simulink model "2025-11-18 - V0.2.6 - FullFMS"  (R2025b)
settings: Solver=VariableStepAuto  StartTime=0.0  StopTime=inf  RelTol=1e-3
libraries: opcualib x8
(part 1 of 3)
settings Model: SimulationMode=accelerator  Creator=guilh  LastModifiedBy=guilh

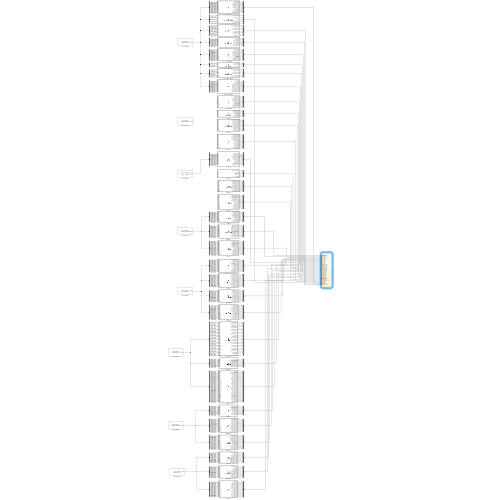
[thumbnail: Simulink's stored preview of the top-level diagram]
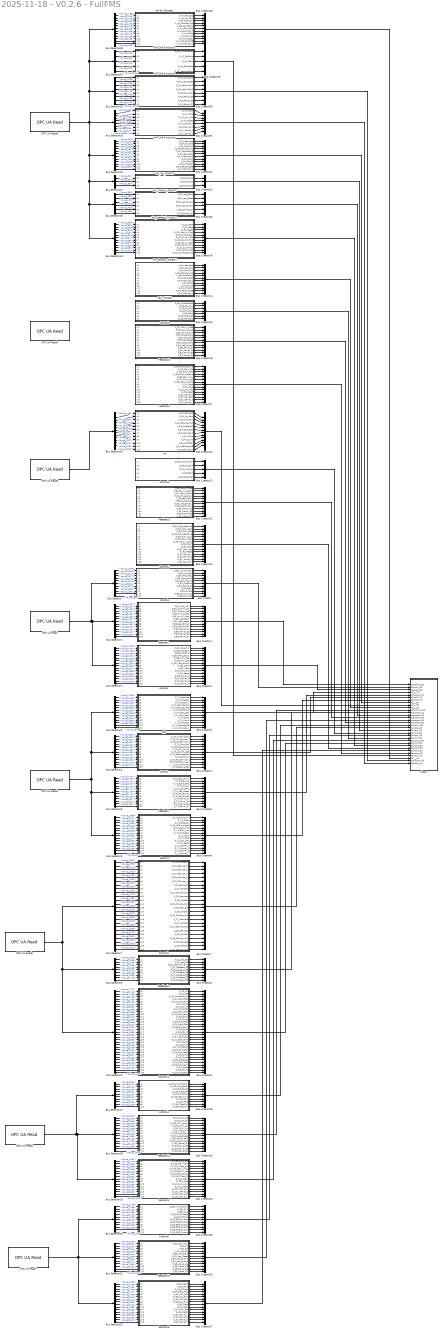
== system 2025-11-18 - V0.2.6 - FullFMS ==
  ASI : MATLAB Function  TreatAsAtomicUnit=on
  Asi : MATLAB Function  TreatAsAtomicUnit=on
  Asi1_HAND2 : MATLAB Function  TreatAsAtomicUnit=on
  Bus Creator : BusCreator  Inputs=11
  Bus Creator1 : BusCreator  Inputs=13
  Bus Creator{5,10,12,14,16,21,24,26,28} (9 alike) : BusCreator  Inputs=12
  Bus Creator11 : BusCreator  Inputs=5
  Bus Creator{2,6,13,17,20} (5 alike) : BusCreator  Inputs=15
  Bus Creator15 : BusCreator  Inputs=7
  Bus Creator18 : BusCreator  Inputs=10
  Bus Creator19 : BusCreator  Inputs=14
  Bus Creator22 : BusCreator  Inputs=3
  Bus Creator23 : BusCreator  Inputs=6
  Bus Creator25 : BusCreator  Inputs=11
  Bus Creator27 : BusCreator  Inputs=16
  Bus Creator29 : BusCreator  Inputs=5
  Bus Creator3 : BusCreator  Inputs=13
  Bus Creator30 : BusCreator  Inputs=8
  Bus Creator31 : BusCreator  Inputs=8
  Bus Creator4 : BusCreator  Inputs=13
  Bus Creator7 : BusCreator  Inputs=24
  Bus Creator8 : BusCreator  Inputs=9
  Bus Creator9 : BusCreator  Inputs=33
  Bus Selector : BusSelector  OutputSignals=Value_1195,Value_1205,Value_1215,Value_1227,Value_1239,Value_1249,Value_1261,Value_1271,Value_1281,Value_1291,Value_1301
  Bus Selector1 : BusSelector  OutputSignals=Value_1317,Value_1327,Value_1337,Value_1347,Value_1357,Value_1367,Value_1377,Value_1387,Value_1397,Value_1407,Value_1417,Value_1427,Value_1437
  Bus Selector10 : BusSelector  OutputSignals=Value_1457,Value_1467,Value_1477,Value_1487,Value_1497,Value_1507,Value_1517,Value_1527,Value_1537,Value_1547,Value_1557,Value_1567
  Bus Selector16 : BusSelector  OutputSignals=Value_215,Value_225,Value_235,Value_245,Value_255,Value_265,Value_275,Value_285,Value_295,Value_305,Value_315,Value_325
  Bus Selector17 : BusSelector  OutputSignals=Value_341,Value_354,Value_367
  Bus Selector18 : BusSelector  OutputSignals=Value_383,Value_393,Value_403,Value_413,Value_423,Value_433
  Bus Selector19 : BusSelector  OutputSignals=Value_569,Value_582,Value_595,Value_608,Value_621,Value_634,Value_647,Value_660,Value_673,Value_686,Value_699,Value_712
  Bus Selector2 : BusSelector  OutputSignals=Value_1458,Value_1471,Value_1486,Value_1499,Value_1512,Value_1525,Value_1538,Value_1551,Value_1564,Value_1577,Value_1590,Value_1603,Value_1616,Value_1629,Value_1642
  Bus Selector20 : BusSelector  OutputSignals=Value_1178,Value_1188,Value_1198,Value_1208,Value_1218,Value_1228,Value_1238,Value_1248,Value_1258,Value_1268,Value_1278
  Bus Selector21 : BusSelector  OutputSignals=Value_1294,Value_1304,Value_1314,Value_1324,Value_1334,Value_1344,Value_1354,Value_1364,Value_1374,Value_1384,Value_1394,Value_1404
  Bus Selector22 : BusSelector  OutputSignals=Value_1423,Value_1436,Value_1451,Value_1464,Value_1477,Value_1490,Value_1503,Value_1516,Value_1529,Value_1542,Value_1555,Value_1568,Value_1581,Value_1594,Value_1607,Value_1620
  Bus Selector23 : BusSelector  OutputSignals=Value_1198,Value_1208,Value_1218,Value_1228,Value_1238,Value_1248,Value_1258,Value_1268,Value_1278,Value_1288,Value_1298,Value_1308
  Bus Selector24 : BusSelector  OutputSignals=Value_1324,Value_1334,Value_1344,Value_1354,Value_1364
  Bus Selector25 : BusSelector  OutputSignals=Value_1380,Value_1390,Value_1400,Value_1410,Value_1420,Value_1430,Value_1440,Value_1450
  Bus Selector26 : BusSelector  OutputSignals=Value_1469,Value_1482,Value_1495,Value_1508,Value_1521,Value_1534,Value_1547,Value_1560
  Bus Selector27 : BusSelector  OutputSignals=Value_1204,Value_1214,Value_1224,Value_1234,Value_1244,Value_1254,Value_1264,Value_1274,Value_1284,Value_1294
  Bus Selector28 : BusSelector  OutputSignals=Value_1310,Value_1320,Value_1330,Value_1340,Value_1350,Value_1360,Value_1370,Value_1380,Value_1390,Value_1400,Value_1410,Value_1420,Value_1430,Value_1440
  Bus Selector29 : BusSelector  OutputSignals=Value_1461,Value_1474,Value_1489,Value_1502,Value_1515,Value_1528,Value_1541,Value_1554,Value_1567,Value_1580,Value_1593,Value_1606,Value_1619,Value_1632,Value_1645
  Bus Selector3 : BusSelector  OutputSignals=Value_1455,Value_1465,Value_1475,Value_1485,Value_1495,Value_1505,Value_1515,Value_1525,Value_1535,Value_1545,Value_1555,Value_1565,Value_1575
  Bus Selector4 : BusSelector  OutputSignals=Value_1591,Value_1601,Value_1611,Value_1621,Value_1631,Value_1641,Value_1651,Value_1661,Value_1671,Value_1681,Value_1691,Value_1701,Value_1711
  Bus Selector5 : BusSelector  OutputSignals=Value_1727,Value_1737,Value_1747,Value_1757,Value_1767,Value_1777,Value_1787,Value_1797,Value_1807,Value_1817,Value_1827,Value_1837
  Bus Selector6 : BusSelector  OutputSignals=Value_1858,Value_1871,Value_1886,Value_1899,Value_1912,Value_1925,Value_1938,Value_1951,Value_1964,Value_1977,Value_1990,Value_2003,Value_2016,Value_2029,Value_2042
  Bus Selector7 : BusSelector  OutputSignals=Value_1382,Value_1392,Value_1402,Value_1412,Value_1422,Value_1432,Value_1442,Value_1452,Value_1462,Value_1472,Value_1482,Value_1492,Value_1502,Value_1512,Value_1522,Value_1532,Value_1542,Value_1552,Value_1562,Value_1572,Value_1582,Value_1592,Value_1602,Value_1612
  Bus Selector8 : BusSelector  OutputSignals=Value_1628,Value_1638,Value_1648,Value_1658,Value_1668,Value_1678,Value_1688,Value_1698,Value_1708
  Bus Selector9 : BusSelector  OutputSignals=Value_1727,Value_1740,Value_1755,Value_1768,Value_1781,Value_1794,Value_1807,Value_1820,Value_1833,Value_1846,Value_1859,Value_1872,Value_1885,Value_1898,Value_1911,Value_1924,Value_1937,Value_1950,Value_1963,Value_1976,Value_1989,Value_2002,Value_2015,Value_2028,Value_2041,Value_2054,Value_2067,Value_2080,Value_2093,Value_2106,Value_2119,Value_2132,Value_2145
  Chart : Stateflow chart  TreatAsAtomicUnit=on
      settings: PortSchema="{\"entries\":[{\"content\":{\"sides\":[{\"content\":{\"connectorIds\":[\"In2\",\"In1\",\"In3\",\"In4\",\"In6\",\"In5\",\"In7\",\"In8\",\"In9\",\"In10\",\"In11\",\"In12\",\"In13\",\"In14\",\"In15\",\"In16\",\"In17\",\"In18\",\"In19\",\"In20\",\"In21\",\"In22\",\"In23\",\"In24\",\"In25\",\"In26\",\"In27\",\"In28\",\"In29\",\"In30\",\"In31\",\"In32\"]},\"type\":\"ConnectorPlacement.EquallySpacedRectSide\",\"uuid\":\"e54bf7d4-7c7d-41d9-a8b8-f479ac319a99\"},{\"content\":{\"side\":\"RIGHT\"},\"type\":\"ConnectorPlacement.EquallySpacedRectSide\",\"uuid\":\"d3c20706-71bd-4e26-b40f-0ee7e71b06ee\"},{\"content\":{\"side\":\"TOP\"},\"type\":\"ConnectorPlacement.EquallySpacedRectSide\",\"uuid\":\"ecfb6920-e95b-4ed8-99f9-df5ce878328e\"}]},\"type\":\"ConnectorPlacement.EquallySpacedConnector\",\"uuid\":\"2e714192-4eea-4e1a-8945-7c827feed48f\"}],\"packageUris\":[\"http://schema.mathworks.com/mf0/Connector/R2020b\"],\"version\":\"1.0\"}"
  Control : MATLAB Function  TreatAsAtomicUnit=on
  Control1 : MATLAB Function  TreatAsAtomicUnit=on
  Control2 : MATLAB Function  TreatAsAtomicUnit=on
  Control3 : MATLAB Function  TreatAsAtomicUnit=on
  Control4 : MATLAB Function  TreatAsAtomicUnit=on
  Control5 : MATLAB Function  TreatAsAtomicUnit=on
  Feedback : MATLAB Function  TreatAsAtomicUnit=on
  Feedback1 : MATLAB Function  TreatAsAtomicUnit=on
  Feedback2 : MATLAB Function  TreatAsAtomicUnit=on
  Feedback3 : MATLAB Function  TreatAsAtomicUnit=on
  Feedback4 : MATLAB Function  TreatAsAtomicUnit=on
  Feedback5 : MATLAB Function  TreatAsAtomicUnit=on
  MATLAB Function1 : MATLAB Function  TreatAsAtomicUnit=on
  MATLAB Function2 : MATLAB Function  TreatAsAtomicUnit=on
  MATLAB Function3 : MATLAB Function  TreatAsAtomicUnit=on
  OPC UA Read : opcualib/OPC UA Read  SelectedServer=AAS OPC Distribution  ServerList=AAS OPC Distribution  NodeList={ '1', 'Value', '6', '1195', '1'; '2', 'Value', '6', '1205', '1'; '3', 'Value', '6', '1215', '1'; '4', 'Value', '6', '1227', '1'; '5', 'Value', '6', '1239', '1'; '6', 'Value', '6', '1249', '1'; '7', 'Value', '6', '1261', '1'; '8', 'Value', '6', '1271', '1'; '9', 'Value', '6', '1281', '1'; '10', 'Value', '6', '1291', '1'; '11', 'Value', '6', '1301', '1'; '12', 'Value', '6', '1317', '1'; '13', 'Value', '6', '1327', '1'; '14', 'Value', '6', '1337', '1'; '15', 'Value', '6', '1347', '1'; '16', 'Value', '6', '1357', '1'; '17', 'Value', '6', '1367', '1'; '18', 'Value', '6', '1377', '1'; '19', 'Value', '6', '1387', '1'; '20', 'Value', '6', '1397', '1'; '21', 'Value', '6', '1407', '1'; '22', 'Value', '6', '1417', '1'; '23', 'Value', '6', '1427', '1'; '24', 'Value', '6', '1437', '1'; '25', 'Value', '6', '1458', '1'; '26', 'Value', '6', '1471', '1'; '27', 'Value', '6', '1486', '1'; '28', 'Value', '6', '1499', '1'; '29', 'Value', '6', '1512', '1'; '30', 'Value', '6', '1525', '1'; '31', 'Value', '6', '1538', '1'; '32', 'Value', '6', '1551', '1'; '33', 'Value', '6', '1564', '1'; '34', 'Value', '6', '1577', '1'; '35', 'Value', '6', '1590', '1'; '36', 'Value', '6', '1603', '1'; '37', 'Value', '6', '1616', '1'; '38', 'Value', '6', '1629', '1'; '39', 'Value', '6', '1642', '1' }  ShowQualityPort=off  ShowTimestampPort=off  ShowTimestampPortAs=Seconds since start  SampleTime=-1
  OPC UA Read1 : opcualib/OPC UA Read  SelectedServer=AAS OPC Testing  ServerList=AAS OPC Testing  NodeList={ '1', 'Value', '6', '1455', '1'; '2', 'Value', '6', '1465', '1'; '3', 'Value', '6', '1475', '1'; '4', 'Value', '6', '1485', '1'; '5', 'Value', '6', '1495', '1'; '6', 'Value', '6', '1505', '1'; '7', 'Value', '6', '1515', '1'; '8', 'Value', '6', '1525', '1'; '9', 'Value', '6', '1535', '1'; '10', 'Value', '6', '1545', '1'; '11', 'Value', '6', '1555', '1'; '12', 'Value', '6', '1565', '1'; '13', 'Value', '6', '1575', '1'; '14', 'Value', '6', '1591', '1'; '15', 'Value', '6', '1601', '1'; '16', 'Value', '6', '1611', '1'; '17', 'Value', '6', '1621', '1'; '18', 'Value', '6', '1631', '1'; '19', 'Value', '6', '1641', '1'; '20', 'Value', '6', '1651', '1'; '21', 'Value', '6', '1661', '1'; '22', 'Value', '6', '1671', '1'; '23', 'Value', '6', '1681', '1'; '24', 'Value', '6', '1691', '1'; '25', 'Value', '6', '1701', '1'; '26', 'Value', '6', '1711', '1'; '27', 'Value', '6', '1727', '1'; '28', 'Value', '6', '1737', '1'; '29', 'Value', '6', '1747', '1'; '30', 'Value', '6', '1757', '1'; '31', 'Value', '6', '1767', '1'; '32', 'Value', '6', '1777', '1'; '33', 'Value', '6', '1787', '1'; '34', 'Value', '6', '1797', '1'; '35', 'Value', '6', '1807', '1'; '36', 'Value', '6', '1817', '1'; '37', 'Value', '6', '1827', '1'; '38', 'Value', '6', '1837', '1'; '39', 'Value', '6', '1858', '1'; '40', 'Value', '6', '1871', '1'; '41', 'Value', '6', '1886', '1'; '42', 'Value', '6', '1899', '1'; '43', 'Value', '6', '1912', '1'; '44', 'Value', '6', '1925', '1'; '45', 'Value', '6', '1938', '1'; '46', 'Value', '6', '1951', '1'; '47', 'Value', '6', '1964', '1'; '48', 'Value', '6', '1977', '1'; '49', 'Value', '6', '1990', '1'; '50', 'Value', '6', '2003', '1'; '51', 'Value', '6', '2016', '1'; '52', 'Value', '6', '2029', '1'; '53', 'Value', '6', '2042', '1' }  ShowQualityPort=off  ShowTimestampPort=off  ShowTimestampPortAs=Seconds since start  SampleTime=-1
  OPC UA Read2 : opcualib/OPC UA Read  SelectedServer=AAS OPC Master  ServerList=AAS OPC Master  NodeList={ '1', 'Value', '6', '1382', '1'; '2', 'Value', '6', '1392', '1'; '3', 'Value', '6', '1402', '1'; '4', 'Value', '6', '1412', '1'; '5', 'Value', '6', '1422', '1'; '6', 'Value', '6', '1432', '1'; '7', 'Value', '6', '1442', '1'; '8', 'Value', '6', '1452', '1'; '9', 'Value', '6', '1462', '1'; '10', 'Value', '6', '1472', '1'; '11', 'Value', '6', '1482', '1'; '12', 'Value', '6', '1492', '1'; '13', 'Value', '6', '1502', '1'; '14', 'Value', '6', '1512', '1'; '15', 'Value', '6', '1522', '1'; '16', 'Value', '6', '1532', '1'; '17', 'Value', '6', '1542', '1'; '18', 'Value', '6', '1552', '1'; '19', 'Value', '6', '1562', '1'; '20', 'Value', '6', '1572', '1'; '21', 'Value', '6', '1582', '1'; '22', 'Value', '6', '1592', '1'; '23', 'Value', '6', '1602', '1'; '24', 'Value', '6', '1612', '1'; '25', 'Value', '6', '1628', '1'; '26', 'Value', '6', '1638', '1'; '27', 'Value', '6', '1648', '1'; '28', 'Value', '6', '1658', '1'; '29', 'Value', '6', '1668', '1'; '30', 'Value', '6', '1678', '1'; '31', 'Value', '6', '1688', '1'; '32', 'Value', '6', '1698', '1'; '33', 'Value', '6', '1708', '1'; '34', 'Value', '6', '1727', '1'; '35', 'Value', '6', '1740', '1'; '36', 'Value', '6', '1755', '1'; '37', 'Value', '6', '1768', '1'; '38', 'Value', '6', '1781', '1'; '39', 'Value', '6', '1794', '1'; '40', 'Value', '6', '1807', '1'; '41', 'Value', '6', '1820', '1'; '42', 'Value', '6', '1833', '1'; '43', 'Value', '6', '1846', '1'; '44', 'Value', '6', '1859', '1'; '45', 'Value', '6', '1872', '1'; '46', 'Value', '6', '1885', '1'; '47', 'Value', '6', '1898', '1'; '48', 'Value', '6', '1911', '1'; '49', 'Value', '6', '1924', '1'; '50', 'Value', '6', '1937', '1'; '51', 'Value', '6', '1950', '1'; '52', 'Value', '6', '1963', '1'; '53', 'Value', '6', '1976', '1'; '54', 'Value', '6', '1989', '1'; '55', 'Value', '6', '2002', '1'; '56', 'Value', '6', '2015', '1'; '57', 'Value', '6', '2028', '1'; '58', 'Value', '6', '2041', '1'; '59', 'Value', '6', '2054', '1'; '60', 'Value', '6', '2067', '1'; '61', 'Value', '6', '2080', '1'; '62', 'Value', '6', '2093', '1'; '63', 'Value', '6', '2106', '1'; '64', 'Value', '6', '2119', '1'; '65', 'Value', '6', '2132', '1'; '66', 'Value', '6', '2145', '1' }  ShowQualityPort=off  ShowTimestampPort=off  ShowTimestampPortAs=Seconds since start  SampleTime=-1
  OPC UA Read3 : opcualib/OPC UA Read  SelectedServer=AAS OPC Handling1  ServerList=AAS OPC Handling1  NodeList={ '1', 'Value', '6', '1457', '1'; '2', 'Value', '6', '1467', '1'; '3', 'Value', '6', '1477', '1'; '4', 'Value', '6', '1487', '1'; '5', 'Value', '6', '1497', '1'; '6', 'Value', '6', '1507', '1'; '7', 'Value', '6', '1517', '1'; '8', 'Value', '6', '1527', '1'; '9', 'Value', '6', '1537', '1'; '10', 'Value', '6', '1547', '1'; '11', 'Value', '6', '1557', '1'; '12', 'Value', '6', '1567', '1' }  ShowQualityPort=off  ShowTimestampPort=off  ShowTimestampPortAs=Seconds since start  SampleTime=-1
  OPC UA Read4 : opcualib/OPC UA Read  SelectedServer=AAS OPC Handling2  ServerList=AAS OPC Handling2  NodeList={ '1', 'Value', '6', '572', '1'; '2', 'Value', '6', '582', '1'; '3', 'Value', '6', '592', '1'; '4', 'Value', '6', '602', '1'; '5', 'Value', '6', '612', '1'; '6', 'Value', '6', '622', '1'; '7', 'Value', '6', '632', '1'; '8', 'Value', '6', '642', '1'; '9', 'Value', '6', '652', '1'; '10', 'Value', '6', '662', '1'; '11', 'Value', '6', '672', '1'; '12', 'Value', '6', '682', '1'; '13', 'Value', '6', '698', '1'; '14', 'Value', '6', '708', '1'; '15', 'Value', '6', '718', '1'; '16', 'Value', '6', '728', '1'; '17', 'Value', '6', '738', '1'; '18', 'Value', '6', '748', '1'; '19', 'Value', '6', '758', '1'; '20', 'Value', '6', '774', '1'; '21', 'Value', '6', '784', '1'; '22', 'Value', '6', '794', '1'; '23', 'Value', '6', '804', '1'; '24', 'Value', '6', '814', '1'; '25', 'Value', '6', '824', '1'; '26', 'Value', '6', '834', '1'; '27', 'Value', '6', '844', '1'; '28', 'Value', '6', '854', '1'; '29', 'Value', '6', '864', '1'; '30', 'Value', '6', '874', '1'; '31', 'Value', '6', '884', '1'; '32', 'Value', '6', '905', '1'; '33', 'Value', '6', '918', '1'; '34', 'Value', '6', '933', '1'; '35', 'Value', '6', '946', '1'; '36', 'Value', '6', '959', '1'; '37', 'Value', '6', '972', '1'; '38', 'Value', '6', '985', '1'; '39', 'Value', '6', '998', '1'; '40', 'Value', '6', '1011', '1'; '41', 'Value', '6', '1024', '1'; '42', 'Value', '6', '1037', '1'; '43', 'Value', '6', '1050', '1'; '44', 'Value', '6', '1063', '1'; '45', 'Value', '6', '1076', '1'; '46', 'Value', '6', '1089', '1' }  ShowQualityPort=off  ShowTimestampPort=off  ShowTimestampPortAs=Seconds since start  SampleTime=-1
  OPC UA Read5 : opcualib/OPC UA Read  SelectedServer=AAS OPC Processing  ServerList=AAS OPC Processing  NodeList={ '1', 'Value', '6', '1204', '1'; '2', 'Value', '6', '1214', '1'; '3', 'Value', '6', '1224', '1'; '4', 'Value', '6', '1234', '1'; '5', 'Value', '6', '1244', '1'; '6', 'Value', '6', '1254', '1'; '7', 'Value', '6', '1264', '1'; '8', 'Value', '6', '1274', '1'; '9', 'Value', '6', '1284', '1'; '10', 'Value', '6', '1294', '1'; '11', 'Value', '6', '1310', '1'; '12', 'Value', '6', '1320', '1'; '13', 'Value', '6', '1330', '1'; '14', 'Value', '6', '1340', '1'; '15', 'Value', '6', '1350', '1'; '16', 'Value', '6', '1360', '1'; '17', 'Value', '6', '1370', '1'; '18', 'Value', '6', '1380', '1'; '19', 'Value', '6', '1390', '1'; '20', 'Value', '6', '1400', '1'; '21', 'Value', '6', '1410', '1'; '22', 'Value', '6', '1420', '1'; '23', 'Value', '6', '1430', '1'; '24', 'Value', '6', '1440', '1'; '25', 'Value', '6', '1461', '1'; '26', 'Value', '6', '1474', '1'; '27', 'Value', '6', '1489', '1'; '28', 'Value', '6', '1502', '1'; '29', 'Value', '6', '1515', '1'; '30', 'Value', '6', '1528', '1'; '31', 'Value', '6', '1541', '1'; '32', 'Value', '6', '1554', '1'; '33', 'Value', '6', '1567', '1'; '34', 'Value', '6', '1580', '1'; '35', 'Value', '6', '1593', '1'; '36', 'Value', '6', '1606', '1'; '37', 'Value', '6', '1619', '1'; '38', 'Value', '6', '1632', '1'; '39', 'Value', '6', '1645', '1' }  ShowQualityPort=off  ShowTimestampPort=off  ShowTimestampPortAs=Seconds since start  SampleTime=-1
  OPC UA Read6 : opcualib/OPC UA Read  SelectedServer=Node-RED OPCUA  ServerList=Node-RED OPCUA  NodeList={ '1', 'Value', '6', '215', '1'; '2', 'Value', '6', '225', '1'; '3', 'Value', '6', '235', '1'; '4', 'Value', '6', '245', '1'; '5', 'Value', '6', '255', '1'; '6', 'Value', '6', '265', '1'; '7', 'Value', '6', '275', '1'; '8', 'Value', '6', '285', '1'; '9', 'Value', '6', '295', '1'; '10', 'Value', '6', '305', '1'; '11', 'Value', '6', '315', '1'; '12', 'Value', '6', '325', '1'; '13', 'Value', '6', '341', '1'; '14', 'Value', '6', '354', '1'; '15', 'Value', '6', '367', '1'; '16', 'Value', '6', '383', '1'; '17', 'Value', '6', '393', '1'; '18', 'Value', '6', '403', '1'; '19', 'Value', '6', '413', '1'; '20', 'Value', '6', '423', '1'; '21', 'Value', '6', '433', '1'; '22', 'Value', '6', '569', '1'; '23', 'Value', '6', '582', '1'; '24', 'Value', '6', '595', '1'; '25', 'Value', '6', '608', '1'; '26', 'Value', '6', '621', '1'; '27', 'Value', '6', '634', '1'; '28', 'Value', '6', '647', '1'; '29', 'Value', '6', '660', '1'; '30', 'Value', '6', '673', '1'; '31', 'Value', '6', '686', '1'; '32', 'Value', '6', '699', '1'; '33', 'Value', '6', '712', '1'; '34', 'Value', '6', '1198', '1'; '35', 'Value', '6', '1208', '1'; '36', 'Value', '6', '1218', '1'; '37', 'Value', '6', '1228', '1'; '38', 'Value', '6', '1238', '1'; '39', 'Value', '6', '1248', '1'; '40', 'Value', '6', '1258', '1'; '41', 'Value', '6', '1268', '1'; '42', 'Value', '6', '1278', '1'; '43', 'Value', '6', '1288', '1'; '44', 'Value', '6', '1298', '1'; '45', 'Value', '6', '1308', '1'; '46', 'Value', '6', '1324', '1'; '47', 'Value', '6', '1334', '1'; '48', 'Value', '6', '1344', '1'; '49', 'Value', '6', '1354', '1'; '50', 'Value', '6', '1364', '1'; '51', 'Value', '6', '1380', '1'; '52', 'Value', '6', '1390', '1'; '53', 'Value', '6', '1400', '1'; '54', 'Value', '6', '1410', '1'; '55', 'Value', '6', '1420', '1'; '56', 'Value', '6', '1430', '1'; '57', 'Value', '6', '1440', '1'; '58', 'Value', '6', '1450', '1'; '59', 'Value', '6', '1469', '1'; '60', 'Value', '6', '1482', '1'; '61', 'Value', '6', '1495', '1'; '62', 'Value', '6', '1508', '1'; '63', 'Value', '6', '1521', '1'; '64', 'Value', '6', '1534', '1'; '65', 'Value', '6', '1547', '1'; '66', 'Value', '6', '1560', '1' }  ShowQualityPort=off  ShowTimestampPort=off  ShowTimestampPortAs=Seconds since start  SampleTime=-1
  OPC UA Read7 : opcualib/OPC UA Read  SelectedServer=AAS OPC Sorting  ServerList=AAS OPC Sorting  NodeList={ '1', 'Value', '6', '1178', '1'; '2', 'Value', '6', '1188', '1'; '3', 'Value', '6', '1198', '1'; '4', 'Value', '6', '1208', '1'; '5', 'Value', '6', '1218', '1'; '6', 'Value', '6', '1228', '1'; '7', 'Value', '6', '1238', '1'; '8', 'Value', '6', '1248', '1'; '9', 'Value', '6', '1258', '1'; '10', 'Value', '6', '1268', '1'; '11', 'Value', '6', '1278', '1'; '12', 'Value', '6', '1294', '1'; '13', 'Value', '6', '1304', '1'; '14', 'Value', '6', '1314', '1'; '15', 'Value', '6', '1324', '1'; '16', 'Value', '6', '1334', '1'; '17', 'Value', '6', '1344', '1'; '18', 'Value', '6', '1354', '1'; '19', 'Value', '6', '1364', '1'; '20', 'Value', '6', '1374', '1'; '21', 'Value', '6', '1384', '1'; '22', 'Value', '6', '1394', '1'; '23', 'Value', '6', '1404', '1'; '24', 'Value', '6', '1423', '1'; '25', 'Value', '6', '1436', '1'; '26', 'Value', '6', '1451', '1'; '27', 'Value', '6', '1464', '1'; '28', 'Value', '6', '1477', '1'; '29', 'Value', '6', '1490', '1'; '30', 'Value', '6', '1503', '1'; '31', 'Value', '6', '1516', '1'; '32', 'Value', '6', '1529', '1'; '33', 'Value', '6', '1542', '1'; '34', 'Value', '6', '1555', '1'; '35', 'Value', '6', '1568', '1'; '36', 'Value', '6', '1581', '1'; '37', 'Value', '6', '1594', '1'; '38', 'Value', '6', '1607', '1'; '39', 'Value', '6', '1620', '1' }  ShowQualityPort=off  ShowTimestampPort=off  ShowTimestampPortAs=Seconds since start  SampleTime=-1
  Sensors : MATLAB Function  TreatAsAtomicUnit=on
  Sensors1 : MATLAB Function  TreatAsAtomicUnit=on
  Sensors2 : MATLAB Function  TreatAsAtomicUnit=on
  Sensors3 : MATLAB Function  TreatAsAtomicUnit=on
  Sensors4 : MATLAB Function  TreatAsAtomicUnit=on
  Sensors5 : MATLAB Function  TreatAsAtomicUnit=on
  controls : MATLAB Function  TreatAsAtomicUnit=on
  fcn Asi Storage : MATLAB Function  TreatAsAtomicUnit=on
  fcn_Asi_ROBOT : MATLAB Function  TreatAsAtomicUnit=on
  fcn_Control_ROBOT : MATLAB Function  TreatAsAtomicUnit=on
  fcn_Feedback_ROBOT : MATLAB Function  TreatAsAtomicUnit=on
  fcn_Sensors_ROBOT : MATLAB Function  TreatAsAtomicUnit=on
  feedback : MATLAB Function  TreatAsAtomicUnit=on
  sensors : MATLAB Function  TreatAsAtomicUnit=on
  wires:
  feedback/1(F_82_Pist_Adv) -> Bus Creator1/1
  feedback/2(F_82_Suction_On) -> Bus Creator1/2
  feedback/3(F_82_Suction_Off) -> Bus Creator1/3
  feedback/4(F_82_Arm_2_Del) -> Bus Creator1/4
  feedback/5(F_82_Arm_2_Mag) -> Bus Creator1/5
  feedback/6(F_83_Led_Start) -> Bus Creator1/6
  feedback/7(F_83_Led_Reset) -> Bus Creator1/7
  feedback/8(F_83_Led_Extra1) -> Bus Creator1/8
  feedback/9(F_83_Led_Extra2) -> Bus Creator1/9
  feedback/10(F_83_Panel_O4) -> Bus Creator1/10
  feedback/11(F_83_Panel_O5) -> Bus Creator1/11
  feedback/12(F_83_Panel_O6) -> Bus Creator1/12
  feedback/13(F_83_Panel_O7) -> Bus Creator1/13
  sensors/1(O_80_Mag_Full) -> Bus Creator2/1
  sensors/2(O_80_Pist_Back) -> Bus Creator2/2
  sensors/3(O_80_Pist_Fwd) -> Bus Creator2/3
  sensors/4(O_80_Part_Stuck) -> Bus Creator2/4
  sensors/5(O_80_Arm_Mag) -> Bus Creator2/5
  sensors/6(O_80_Arm_Del) -> Bus Creator2/6
  sensors/7(O_80_Mag_Empty) -> Bus Creator2/7
  sensors/8(O_81_Start) -> Bus Creator2/8
  sensors/9(O_81_Stop) -> Bus Creator2/9
  sensors/10(O_81_Key_Pos) -> Bus Creator2/10
  sensors/11(O_81_Reset) -> Bus Creator2/11
  sensors/12(O_81_Panel_I4) -> Bus Creator2/12
  sensors/13(O_81_Panel_I5) -> Bus Creator2/13
  sensors/14(O_81_Panel_I6) -> Bus Creator2/14
  sensors/15(O_81_Panel_I7) -> Bus Creator2/15
  ASI/1(A_74_Request) -> Bus Creator3/1
  ASI/2(A_74_No_Cart) -> Bus Creator3/2
  ASI/3(A_74_Cart_Full) -> Bus Creator3/3
  ASI/4(A_74_CRoute_Out) -> Bus Creator3/4
  ASI/5(A_74_CRoute_In80) -> Bus Creator3/5
  ASI/6(A_73_TestCartID) -> Bus Creator3/6
  ASI/7(A_74_Cart_Stat) -> Bus Creator3/7
  ASI/8(A_74_Cart_Next) -> Bus Creator3/8
  ASI/9(A_74_Optic) -> Bus Creator3/9
  ASI/10(A_74_Count) -> Bus Creator3/10
  ASI/11(A_74_Pist_Bck) -> Bus Creator3/11
  ASI/12(A_74_Release_FB) -> Bus Creator3/12
  ASI/13(A_74_CRoute_In) -> Bus Creator3/13
  Control/1(C_75_Initialization) -> Bus Creator4/1
  Control/2(C_75_ID_Delivery1) -> Bus Creator4/2
  Control/3(C_75_ID_Delivery2) -> Bus Creator4/3
  Control/4(C_75_Part_Del) -> Bus Creator4/4
  Control/5(C_75_RQ_Part_Del) -> Bus Creator4/5
  Control/6(C_75_RQ_Wrong) -> Bus Creator4/6
  Control/7(C_75_Identified80) -> Bus Creator4/7
  Control/8(C_75_Requested80) -> Bus Creator4/8
  Control/9(C_72_Profibus) -> Bus Creator4/9
  Control/10(C_75_RQ_Delivery1) -> Bus Creator4/10
  Control/11(C_75_RQ_Delivery2) -> Bus Creator4/11
  Control/12(C_75_Identified) -> Bus Creator4/12
  Control/13(C_75_Requested) -> Bus Creator4/13
  Feedback/1(F_72_Elev_Down) -> Bus Creator5/1
  Feedback/2(F_72_Elev_Up) -> Bus Creator5/2
  Feedback/3(F_72_Eject_Part) -> Bus Creator5/3
  Feedback/4(F_72_Air_On) -> Bus Creator5/4
  Feedback/5(F_73_Led_Start) -> Bus Creator5/5
  Feedback/6(F_73_Led_Reset) -> Bus Creator5/6
  Feedback/7(F_73_Led_Extra1) -> Bus Creator5/7
  Feedback/8(F_73_Led_Extra2) -> Bus Creator5/8
  Feedback/9(F_73_Panel_O4) -> Bus Creator5/9
  Feedback/10(F_73_Panel_O5) -> Bus Creator5/10
  Feedback/11(F_73_Panel_O6) -> Bus Creator5/11
  Feedback/12(F_73_Panel_O7) -> Bus Creator5/12
  Sensors/1(O_70_SInductive) -> Bus Creator6/1
  Sensors/2(O_70_SPart) -> Bus Creator6/2
  Sensors/3(O_70_SStation) -> Bus Creator6/3
  Sensors/4(O_70_SPart_Height) -> Bus Creator6/4
  Sensors/5(O_70_Elev_High) -> Bus Creator6/5
  Sensors/6(O_70_Elev_Low) -> Bus Creator6/6
  Sensors/7(O_70_Pist_Back) -> Bus Creator6/7
  Sensors/8(O_71_Start) -> Bus Creator6/8
  Sensors/9(O_71_Stop) -> Bus Creator6/9
  Sensors/10(O_71_Key_Pos) -> Bus Creator6/10
  Sensors/11(O_71_Reset) -> Bus Creator6/11
  Sensors/12(O_71_Panel_I4) -> Bus Creator6/12
  Sensors/13(O_71_Panel_I5) -> Bus Creator6/13
  Sensors/14(O_71_Panel_I6) -> Bus Creator6/14
  Sensors/15(O_71_Panel_I7) -> Bus Creator6/15
  Bus Creator/1 -> Chart/1(Control_80)
  Bus Creator1/1 -> Chart/2(Actuators_80)
  Bus Creator2/1 -> Chart/3(Sensors_80)
  Bus Creator6/1 -> Chart/7(Sensors_70)
  Bus Creator5/1 -> Chart/6(Actuators_70)
  Bus Creator4/1 -> Chart/5(Control_70)
  Bus Creator3/1 -> Chart/4(AS_i_70)
  Control1/1(C_24_CRoute_In) -> Bus Creator7/1
  Control1/2(C_25_CRoute_In) -> Bus Creator7/2
  Control1/3(C_26_CRoute_In) -> Bus Creator7/3
  Control1/4(C_27_CRoute_In) -> Bus Creator7/4
  Control1/5(C_28_CRoute_In) -> Bus Creator7/5
  Control1/6(C_29_CRoute_In) -> Bus Creator7/6
  Control1/7(C_24_Request) -> Bus Creator7/7
  Control1/8(C_24_CartDel) -> Bus Creator7/8
  Control1/9(C_24_CRoute_Out) -> Bus Creator7/9
  Control1/10(C_25_Request) -> Bus Creator7/10
  Control1/11(C_25_CartDel) -> Bus Creator7/11
  Control1/12(C_25_CRoute_Out) -> Bus Creator7/12
  Control1/13(C_26_Request) -> Bus Creator7/13
  Control1/14(C_26_CartDel) -> Bus Creator7/14
  Control1/15(C_26_CRoute_Out) -> Bus Creator7/15
  Control1/16(C_27_Request) -> Bus Creator7/16
  Control1/17(C_27_CartDel) -> Bus Creator7/17
  Control1/18(C_27_CRoute_Out) -> Bus Creator7/18
  Control1/19(C_28_Request) -> Bus Creator7/19
  Control1/20(C_28_CartDel) -> Bus Creator7/20
  Control1/21(C_28_CRoute_Out) -> Bus Creator7/21
  Control1/22(C_29_Request) -> Bus Creator7/22
  Control1/23(C_29_CartDel) -> Bus Creator7/23
  Control1/24(C_29_CRoute_Out) -> Bus Creator7/24
  Feedback1/1(F_22_Led_On) -> Bus Creator8/1
  Feedback1/2(F_22_Led_Off) -> Bus Creator8/2
  Feedback1/3(F_22_Led_Conveyor) -> Bus Creator8/3
  Feedback1/4(F_24_Release_FB) -> Bus Creator8/4
  Feedback1/5(F_25_Release_FB) -> Bus Creator8/5
  Feedback1/6(F_26_Release_FB) -> Bus Creator8/6
  Feedback1/7(F_27_Release_FB) -> Bus Creator8/7
  Feedback1/8(F_28_Release_FB) -> Bus Creator8/8
  Feedback1/9(F_29_Release_FB) -> Bus Creator8/9
  Sensors1/1(O_20_On) -> Bus Creator9/1
  Sensors1/2(O_20_Off) -> Bus Creator9/2
  Sensors1/3(O_20_Controler_On) -> Bus Creator9/3
  Sensors1/4(O_24_Cart_Stat) -> Bus Creator9/4
  Sensors1/5(O_24_Cart_Next) -> Bus Creator9/5
  Sensors1/6(O_24_Optic) -> Bus Creator9/6
  Sensors1/7(O_24_Count) -> Bus Creator9/7
  Sensors1/8(O_24_Pist_Bck) -> Bus Creator9/8
  Sensors1/9(O_25_Cart_Stat) -> Bus Creator9/9
  Sensors1/10(O_25_Cart_Next) -> Bus Creator9/10
  Sensors1/11(O_25_Optic) -> Bus Creator9/11
  Sensors1/12(O_25_Count) -> Bus Creator9/12
  Sensors1/13(O_25_Pist_Back) -> Bus Creator9/13
  Sensors1/14(O_26_Cart_Stat) -> Bus Creator9/14
  Sensors1/15(O_26_Cart_Next) -> Bus Creator9/15
  Sensors1/16(O_26_Optic) -> Bus Creator9/16
  Sensors1/17(O_26_Count) -> Bus Creator9/17
  Sensors1/18(O_26_Pist_Back) -> Bus Creator9/18
  Sensors1/19(O_27_Cart_Stat) -> Bus Creator9/19
  Sensors1/20(O_27_Cart_Next) -> Bus Creator9/20
  Sensors1/21(O_27_Optic) -> Bus Creator9/21
  Sensors1/22(O_27_Count) -> Bus Creator9/22
  Sensors1/23(O_27_Pist_Back) -> Bus Creator9/23
  Sensors1/24(O_28_Cart_Stat) -> Bus Creator9/24
  Sensors1/25(O_28_Cart_Next) -> Bus Creator9/25
  Sensors1/26(O_28_Optic) -> Bus Creator9/26
  Sensors1/27(O_28_Count) -> Bus Creator9/27
  Sensors1/28(O_28_Pist_Back) -> Bus Creator9/28
  Sensors1/29(O_29_Cart_Stat) -> Bus Creator9/29
  Sensors1/30(O_29_Cart_Next) -> Bus Creator9/30
  Sensors1/31(O_29_Optic) -> Bus Creator9/31
  Sensors1/32(O_29_Count) -> Bus Creator9/32
  Sensors1/33(O_29_Pist_Back) -> Bus Creator9/33
  Bus Creator7/1 -> Chart/18(Control_20)
  Bus Creator8/1 -> Chart/12(Actuators_20)
  Bus Creator9/1 -> Chart/24(Sensors_20)
  Sensors2/1(O_50_Part_Reserve) -> Bus Creator13/1
  Sensors2/2(O_50_Claw_Cart) -> Bus Creator13/2
  Sensors2/3(O_50_Claw_Del) -> Bus Creator13/3
  Sensors2/4(O_50_Claw_Reserve) -> Bus Creator13/4
  Sensors2/5(O_50_Claw_Low) -> Bus Creator13/5
  Sensors2/6(O_50_Claw_High) -> Bus Creator13/6
  Sensors2/7(O_50_Part_in_Claw) -> Bus Creator13/7
  Sensors2/8(O_51_Start) -> Bus Creator13/8
  Sensors2/9(O_51_Stop) -> Bus Creator13/9
  Sensors2/10(O_51_Key_Pos) -> Bus Creator13/10
  Sensors2/11(O_51_Reset) -> Bus Creator13/11
  Sensors2/12(O_51_Panel_I4) -> Bus Creator13/12
  Sensors2/13(O_51_Panel_I5) -> Bus Creator13/13
  Sensors2/14(O_51_Panel_I6) -> Bus Creator13/14
  Sensors2/15(O_51_Panel_I7) -> Bus Creator13/15
  Feedback2/1(F_52_Claw_2_Del) -> Bus Creator12/1
  Feedback2/2(F_52_Claw_2_Cart) -> Bus Creator12/2
  Feedback2/3(F_52_Claw_Down) -> Bus Creator12/3
  Feedback2/4(F_52_Close_Claw) -> Bus Creator12/4
  Feedback2/5(F_53_Led_Start) -> Bus Creator12/5
  Feedback2/6(F_53_Led_Reset) -> Bus Creator12/6
  Feedback2/7(F_53_Led_Extra1) -> Bus Creator12/7
  Feedback2/8(F_53_Led_Extra2) -> Bus Creator12/8
  Feedback2/9(F_53_Panel_O4) -> Bus Creator12/9
  Feedback2/10(F_53_Panel_O5) -> Bus Creator12/10
  Feedback2/11(F_53_Panel_O6) -> Bus Creator12/11
  Feedback2/12(F_53_Panel_O7) -> Bus Creator12/12
  Control2/1(C_55_Initialization) -> Bus Creator11/1
  Control2/2(C_55_PD_Sort) -> Bus Creator11/2
  Control2/3(C_52_Profibus) -> Bus Creator11/3
  Control2/4(C_55_Start) -> Bus Creator11/4
  Control2/5(C_55_Cart2Del) -> Bus Creator11/5
  Bus Creator10/1 -> Chart/9(AS_i_50)
  Bus Creator11/1 -> Chart/20(Control_50)
  Bus Creator12/1 -> Chart/14(Actuators_50)
  Bus Creator13/1 -> Chart/26(Sensors_50)
  Asi1_HAND2/1(A_94_Request) -> Bus Creator14/1
  Asi1_HAND2/2(A_94_No_Cart) -> Bus Creator14/2
  Asi1_HAND2/3(A_94_Cart_Full) -> Bus Creator14/3
  Asi1_HAND2/4(A_94_CRoute_Out) -> Bus Creator14/4
  Asi1_HAND2/5(A_93_ProcCartID) -> Bus Creator14/5
  Asi1_HAND2/6(A_94_Cart_Stat) -> Bus Creator14/6
  Asi1_HAND2/7(A_94_Cart_Next) -> Bus Creator14/7
  Asi1_HAND2/8(A_94_Optic) -> Bus Creator14/8
  Asi1_HAND2/9(A_94_Count) -> Bus Creator14/9
  Asi1_HAND2/10(A_94_Pist_Bck) -> Bus Creator14/10
  Asi1_HAND2/11(A_94_Release_FB) -> Bus Creator14/11
  Asi1_HAND2/12(A_94_CRoute_In) -> Bus Creator14/12
  Control3/1(C_95_Initialization) -> Bus Creator15/1
  Control3/2(C_95_PD_Proc) -> Bus Creator15/2
  Control3/3(C_95_PD_Cart) -> Bus Creator15/3
  Control3/4(C_92_Profibus) -> Bus Creator15/4
  Control3/5(C_95_Start) -> Bus Creator15/5
  Control3/6(C_95_Cart2Del) -> Bus Creator15/6
  Control3/7(C_95_Del2Cart) -> Bus Creator15/7
  Feedback3/1(F_92_Claw_2_Cart) -> Bus Creator16/1
  Feedback3/2(F_92_Claw_2_Del) -> Bus Creator16/2
  Feedback3/3(F_92_Claw_Down) -> Bus Creator16/3
  Feedback3/4(F_92_Close_Claw) -> Bus Creator16/4
  Feedback3/5(F_93_Led_Start) -> Bus Creator16/5
  Feedback3/6(F_93_Led_Reset) -> Bus Creator16/6
  Feedback3/7(F_93_Led_Extra1) -> Bus Creator16/7
  Feedback3/8(F_93_Led_Extra2) -> Bus Creator16/8
  Feedback3/9(F_93_Panel_O4) -> Bus Creator16/9
  Feedback3/10(F_93_Panel_O5) -> Bus Creator16/10
  Feedback3/11(F_93_Panel_O6) -> Bus Creator16/11
  Feedback3/12(F_93_Panel_O7) -> Bus Creator16/12
  Sensors3/1(O_90_Part_Reserve) -> Bus Creator17/1
  Sensors3/2(O_90_Claw_Del) -> Bus Creator17/2
  Sensors3/3(O_90_Claw_Cart) -> Bus Creator17/3
  Sensors3/4(O_90_Claw_Reserve) -> Bus Creator17/4
  Sensors3/5(O_90_Claw_Low) -> Bus Creator17/5
  Sensors3/6(O_90_Claw_High) -> Bus Creator17/6
  Sensors3/7(O_90_Part_in_Claw) -> Bus Creator17/7
  Sensors3/8(O_91_Start) -> Bus Creator17/8
  Sensors3/9(O_91_Stop) -> Bus Creator17/9
  Sensors3/10(O_91_Key_Pos) -> Bus Creator17/10
  Sensors3/11(O_91_Reset) -> Bus Creator17/11
  Sensors3/12(O_91_Panel_I4) -> Bus Creator17/12
  Sensors3/13(O_91_Panel_I5) -> Bus Creator17/13
  Sensors3/14(O_91_Panel_I6) -> Bus Creator17/14
  Sensors3/15(O_91_Panel_I7) -> Bus Creator17/15
  Bus Creator14/1 -> Chart/10(AS_i_90)
  Bus Creator15/1 -> Chart/22(Control_90)
  Bus Creator16/1 -> Chart/16(Actuators_90)
  Bus Creator17/1 -> Chart/28(Sensors_90)
  Sensors4/1(O_100_PInit_Pos) -> Bus Creator20/1
  Sensors4/2(O_100_PDrill_Pos) -> Bus Creator20/2
  Sensors4/3(O_100_PTest_Pos) -> Bus Creator20/3
  Sensors4/4(O_100_SDrill_High) -> Bus Creator20/4
  Sensors4/5(O_100_SDrill_Low) -> Bus Creator20/5
  Sensors4/6(O_100_RT_Sensor) -> Bus Creator20/6
  Sensors4/7(O_100_PTest_Ok) -> Bus Creator20/7
  Sensors4/8(O_101_Start) -> Bus Creator20/8
  Sensors4/9(O_101_Stop) -> Bus Creator20/9
  Sensors4/10(O_101_Key_Pos) -> Bus Creator20/10
  Sensors4/11(O_101_Reset) -> Bus Creator20/11
  Sensors4/12(O_101_Panel_I4) -> Bus Creator20/12
  Sensors4/13(O_101_Panel_I5) -> Bus Creator20/13
  Sensors4/14(O_101_Panel_I6) -> Bus Creator20/14
  Sensors4/15(O_101_Panel_I7) -> Bus Creator20/15
  Control4/1(C_105_Initialization) -> Bus Creator18/1
  Control4/2(C_105_Part_ready) -> Bus Creator18/2
  Control4/3(C_105_Test_Ok) -> Bus Creator18/3
  Control4/4(C_105_Test_Fail) -> Bus Creator18/4
  Control4/5(C_102_Profibus) -> Bus Creator18/5
  Control4/6(C_103_RQ_Turns) -> Bus Creator18/6
  Control4/7(C_105_Start) -> Bus Creator18/7
  Control4/8(C_105_Test) -> Bus Creator18/8
  Control4/9(C_105_TestDrill) -> Bus Creator18/9
  Control4/10(C_105_Rotation) -> Bus Creator18/10
  Feedback4/1(F_102_Drill_On) -> Bus Creator19/1
  Feedback4/2(F_102_RT_On) -> Bus Creator19/2
  Feedback4/3(F_102_Drill_Down) -> Bus Creator19/3
  Feedback4/4(F_102_Drill_Up) -> Bus Creator19/4
  Feedback4/5(F_102_Drill_Pin) -> Bus Creator19/5
  Feedback4/6(F_102_Test_Pin) -> Bus Creator19/6
  Feedback4/7(F_103_Led_Start) -> Bus Creator19/7
  Feedback4/8(F_103_Led_Reset) -> Bus Creator19/8
  Feedback4/9(F_103_Led_Extra1) -> Bus Creator19/9
  Feedback4/10(F_103_Led_Extra2) -> Bus Creator19/10
  Feedback4/11(F_103_Panel_O4) -> Bus Creator19/11
  Feedback4/12(F_103_Panel_O5) -> Bus Creator19/12
  Feedback4/13(F_103_Panel_O6) -> Bus Creator19/13
  Feedback4/14(F_103_Panel_O7) -> Bus Creator19/14
  Bus Creator18/1 -> Chart/17(Control_100)
  Bus Creator19/1 -> Chart/11(Actuators_100)
  Bus Creator20/1 -> Chart/23(Sensors_100)
  OPC UA Read6/1 -> Bus Selector19/1, Bus Selector18/1, Bus Selector17/1, Bus Selector16/1, Bus Selector23/1, Bus Selector24/1, Bus Selector25/1, Bus Selector26/1
  Bus Selector16/1 -> fcn_Asi_ROBOT/1(u1)  "<Value_215>"
  Bus Selector16/2 -> fcn_Asi_ROBOT/2(u2)  "<Value_225>"
  Bus Selector16/3 -> fcn_Asi_ROBOT/3(u3)  "<Value_235>"
  Bus Selector16/4 -> fcn_Asi_ROBOT/4(u4)  "<Value_245>"
  Bus Selector16/5 -> fcn_Asi_ROBOT/5(u5)  "<Value_255>"
  Bus Selector16/6 -> fcn_Asi_ROBOT/6(u6)  "<Value_265>"
  Bus Selector16/7 -> fcn_Asi_ROBOT/7(u7)  "<Value_275>"
  Bus Selector16/8 -> fcn_Asi_ROBOT/8(u8)  "<Value_285>"
  Bus Selector16/9 -> fcn_Asi_ROBOT/9(u9)  "<Value_295>"
  Bus Selector16/10 -> fcn_Asi_ROBOT/10(u10)  "<Value_305>"
  Bus Selector16/11 -> fcn_Asi_ROBOT/11(u11)  "<Value_315>"
  Bus Selector16/12 -> fcn_Asi_ROBOT/12(u12)  "<Value_325>"
  Bus Selector17/1 -> fcn_Control_ROBOT/1(u1)  "<Value_341>"
  Bus Selector17/2 -> fcn_Control_ROBOT/2(u2)  "<Value_354>"
  Bus Selector17/3 -> fcn_Control_ROBOT/3(u3)  "<Value_367>"
  Bus Selector18/1 -> fcn_Feedback_ROBOT/1(u1)  "<Value_383>"
  Bus Selector18/2 -> fcn_Feedback_ROBOT/2(u2)  "<Value_393>"
  Bus Selector18/3 -> fcn_Feedback_ROBOT/3(u3)  "<Value_403>"
  Bus Selector18/4 -> fcn_Feedback_ROBOT/4(u4)  "<Value_413>"
  Bus Selector18/5 -> fcn_Feedback_ROBOT/5(u5)  "<Value_423>"
  Bus Selector18/6 -> fcn_Feedback_ROBOT/6(u6)  "<Value_433>"
  fcn_Asi_ROBOT/1(A_34_Request) -> Bus Creator21/1
  fcn_Asi_ROBOT/2(A_34_No_Cart) -> Bus Creator21/2
  fcn_Asi_ROBOT/3(A_34_Cart_Full) -> Bus Creator21/3
  fcn_Asi_ROBOT/4(A_34_CRoute_Out) -> Bus Creator21/4
  fcn_Asi_ROBOT/5(A_32_RoboCartID) -> Bus Creator21/5
  fcn_Asi_ROBOT/6(A_34_Cart_Stat) -> Bus Creator21/6
  fcn_Asi_ROBOT/7(A_34_Cart_Next) -> Bus Creator21/7
  fcn_Asi_ROBOT/8(A_34_Optic) -> Bus Creator21/8
  fcn_Asi_ROBOT/9(A_34_Count) -> Bus Creator21/9
  fcn_Asi_ROBOT/10(A_34_Pist_Bck) -> Bus Creator21/10
  fcn_Asi_ROBOT/11(A_34_Release_FB) -> Bus Creator21/11
  fcn_Asi_ROBOT/12(A_34_CRoute_In) -> Bus Creator21/12
  fcn_Control_ROBOT/1(C_30_Robot1) -> Bus Creator22/1
  fcn_Control_ROBOT/2(C_30_Robot2) -> Bus Creator22/2
  fcn_Control_ROBOT/3(C_35_Part_Del) -> Bus Creator22/3
  fcn_Feedback_ROBOT/1(F_33_Led_Start) -> Bus Creator23/1
  fcn_Feedback_ROBOT/2(F_33_Led_Reset) -> Bus Creator23/2
  fcn_Feedback_ROBOT/3(F_33_Led_Extra1) -> Bus Creator23/3
  fcn_Feedback_ROBOT/4(F_33_Led_Extra2) -> Bus Creator23/4
  fcn_Feedback_ROBOT/5(F_33_Spring_Cyl) -> Bus Creator23/5
  fcn_Feedback_ROBOT/6(F_33_Cover_Cyl) -> Bus Creator23/6
  fcn_Sensors_ROBOT/1(O_31_Start) -> Bus Creator24/1
  fcn_Sensors_ROBOT/2(O_31_Stop) -> Bus Creator24/2
  fcn_Sensors_ROBOT/3(O_31_Reset) -> Bus Creator24/3
  fcn_Sensors_ROBOT/4(O_31_Part_in_Claw) -> Bus Creator24/4
  fcn_Sensors_ROBOT/5(O_31_Orientation) -> Bus Creator24/5
  fcn_Sensors_ROBOT/6(O_32_Sp_Cyl_Bck) -> Bus Creator24/6
  fcn_Sensors_ROBOT/7(O_32_Sp_Cyl_Fwd) -> Bus Creator24/7
  fcn_Sensors_ROBOT/8(O_32_Co_Cyl_Bck) -> Bus Creator24/8
  fcn_Sensors_ROBOT/9(O_32_Co_Cyl_Fwd) -> Bus Creator24/9
  fcn_Sensors_ROBOT/10(O_32_Sp_PickUp) -> Bus Creator24/10
  fcn_Sensors_ROBOT/11(O_32_Co_PickUp) -> Bus Creator24/11
  fcn_Sensors_ROBOT/12(O_32_CoMag_Empty) -> Bus Creator24/12
  Bus Creator21/1 -> Chart/8(AS_i_30)
  Bus Creator22/1 -> Chart/19(Control_30)
  Bus Creator23/1 -> Chart/13(Actuators_30)
  Bus Creator24/1 -> Chart/25(Sensors_30)
  Control5/1(C_65_Initialization) -> Bus Creator25/1
  Control5/2(C_65_ID_1) -> Bus Creator25/2
  Control5/3(C_65_ID_2) -> Bus Creator25/3
  Control5/4(C_65_Part_Sorted) -> Bus Creator25/4
  Control5/5(C_62_Profibus) -> Bus Creator25/5
  Control5/6(C_65_RBS_Output) -> Bus Creator25/6
  Control5/7(C_65_RSB_Output) -> Bus Creator25/7
  Control5/8(C_65_BRS_Output) -> Bus Creator25/8
  Control5/9(C_65_BSR_Output) -> Bus Creator25/9
  Control5/10(C_65_SRB_Output) -> Bus Creator25/10
  Control5/11(C_65_SBR_Output) -> Bus Creator25/11
  Feedback5/1(F_62_Conveyor) -> Bus Creator26/1
  Feedback5/2(F_62_P1) -> Bus Creator26/2
  Feedback5/3(F_62_P2) -> Bus Creator26/3
  Feedback5/4(F_62_Identify) -> Bus Creator26/4
  Feedback5/5(F_63_Led_Start) -> Bus Creator26/5
  Feedback5/6(F_63_Led_Reset) -> Bus Creator26/6
  Feedback5/7(F_63_Led_Extra1) -> Bus Creator26/7
  Feedback5/8(F_63_Led_Extra2) -> Bus Creator26/8
  Feedback5/9(F_63_Panel_O4) -> Bus Creator26/9
  Feedback5/10(F_63_Panel_O5) -> Bus Creator26/10
  Feedback5/11(F_63_Panel_O6) -> Bus Creator26/11
  Feedback5/12(F_63_Panel_O7) -> Bus Creator26/12
  Sensors5/1(O_60_SPart) -> Bus Creator27/1
  Sensors5/2(O_60_Slnd) -> Bus Creator27/2
  Sensors5/3(O_60_SPhoto) -> Bus Creator27/3
  Sensors5/4(O_60_Part_Pass) -> Bus Creator27/4
  Sensors5/5(O_60_SL1_Bck) -> Bus Creator27/5
  Sensors5/6(O_60_SL1_Fwd) -> Bus Creator27/6
  Sensors5/7(O_60_SL2_Bck) -> Bus Creator27/7
  Sensors5/8(O_60_SL2_Fwd) -> Bus Creator27/8
  Sensors5/9(O_61_Start) -> Bus Creator27/9
  Sensors5/10(O_61_Stop) -> Bus Creator27/10
  Sensors5/11(O_61_Key_Pos) -> Bus Creator27/11
  Sensors5/12(O_61_Reset) -> Bus Creator27/12
  Sensors5/13(O_61_Panel_I4) -> Bus Creator27/13
  Sensors5/14(O_61_Panel_I5) -> Bus Creator27/14
  Sensors5/15(O_61_Panel_I6) -> Bus Creator27/15
  Sensors5/16(O_61_Panel_I7) -> Bus Creator27/16
  Bus Creator25/1 -> Chart/21(Control_60)
  Bus Creator26/1 -> Chart/15(Actuators_60)
  Bus Creator27/1 -> Chart/27(Sensors_60)
  Bus Selector19/1 -> fcn_Sensors_ROBOT/1(u1)  "<Value_569>"
  Bus Selector19/2 -> fcn_Sensors_ROBOT/2(u2)  "<Value_582>"
  Bus Selector19/3 -> fcn_Sensors_ROBOT/3(u3)  "<Value_595>"
  Bus Selector19/4 -> fcn_Sensors_ROBOT/4(u4)  "<Value_608>"
  Bus Selector19/5 -> fcn_Sensors_ROBOT/5(u5)  "<Value_621>"
  Bus Selector19/6 -> fcn_Sensors_ROBOT/6(u6)  "<Value_634>"
  Bus Selector19/7 -> fcn_Sensors_ROBOT/7(u7)  "<Value_647>"
  Bus Selector19/8 -> fcn_Sensors_ROBOT/8(u8)  "<Value_660>"
  Bus Selector19/9 -> fcn_Sensors_ROBOT/9(u9)  "<Value_673>"
  Bus Selector19/10 -> fcn_Sensors_ROBOT/10(u10)  "<Value_686>"
  Bus Selector19/11 -> fcn_Sensors_ROBOT/11(u11)  "<Value_699>"
  Bus Selector19/12 -> fcn_Sensors_ROBOT/12(u12)  "<Value_712>"
  MATLAB Function1/1(C_45_Initialization) -> Bus Creator29/1
  MATLAB Function1/2(C_42_Profibus) -> Bus Creator29/2
  MATLAB Function1/3(C_45_Start) -> Bus Creator29/3
  MATLAB Function1/4(C_45_StorePart) -> Bus Creator29/4
  MATLAB Function1/5(C_45_RetrievePart) -> Bus Creator29/5
  MATLAB Function2/1(F_43_Led_Start) -> Bus Creator30/1
  MATLAB Function2/2(F_43_Led_Reset) -> Bus Creator30/2
  MATLAB Function2/3(F_43_Led_Extra1) -> Bus Creator30/3
  MATLAB Function2/4(F_43_Led_Extra2) -> Bus Creator30/4
  MATLAB Function2/5(F_43_Panel_O4) -> Bus Creator30/5
  MATLAB Function2/6(F_43_Panel_O5) -> Bus Creator30/6
  MATLAB Function2/7(F_43_Panel_O6) -> Bus Creator30/7
  MATLAB Function2/8(F_43_Panel_O7) -> Bus Creator30/8
  MATLAB Function3/1(O_41_Start) -> Bus Creator31/1
  MATLAB Function3/2(O_41_Stop) -> Bus Creator31/2
  MATLAB Function3/3(O_41_Key_Pos) -> Bus Creator31/3
  MATLAB Function3/4(O_41_Reset) -> Bus Creator31/4
  MATLAB Function3/5(O_41_Panel_I4) -> Bus Creator31/5
  MATLAB Function3/6(O_41_Panel_I5) -> Bus Creator31/6
  MATLAB Function3/7(O_41_Panel_I6) -> Bus Creator31/7
  MATLAB Function3/8(O_41_Panel_I7) -> Bus Creator31/8
  Bus Creator28/1 -> Chart/30(AS_i_40)
  Bus Creator29/1 -> Chart/29(Control_40)
  Bus Creator30/1 -> Chart/31(Actuators_40)
  Bus Creator31/1 -> Chart/32(Sensors_40)
  fcn Asi Storage/7(A_44_Cart_Next) -> Bus Creator28/7
  fcn Asi Storage/1(A_44_Request) -> Bus Creator28/1
  fcn Asi Storage/2(A_44_No_Cart) -> Bus Creator28/2
  fcn Asi Storage/3(A_44_Cart_Full) -> Bus Creator28/3
  fcn Asi Storage/4(A_44_CRoute_Out) -> Bus Creator28/4
  fcn Asi Storage/5(A_43_StorCartID) -> Bus Creator28/5
  fcn Asi Storage/6(A_44_Cart_Stat) -> Bus Creator28/6
  fcn Asi Storage/8(A_44_Optic) -> Bus Creator28/8
  fcn Asi Storage/9(A_44_Count) -> Bus Creator28/9
  fcn Asi Storage/10(A_44_Pist_Bck) -> Bus Creator28/10
  fcn Asi Storage/11(A_44_Release_FB) -> Bus Creator28/11
  fcn Asi Storage/12(A_44_CRoute_In) -> Bus Creator28/12
  Bus Selector23/1 -> fcn Asi Storage/1(u1)  "<Value_1198>"
  Bus Selector23/2 -> fcn Asi Storage/2(u2)  "<Value_1208>"
  Bus Selector23/3 -> fcn Asi Storage/3(u3)  "<Value_1218>"
  Bus Selector23/4 -> fcn Asi Storage/4(u4)  "<Value_1228>"
  Bus Selector23/5 -> fcn Asi Storage/5(u5)  "<Value_1238>"
  Bus Selector23/6 -> fcn Asi Storage/6(u6)  "<Value_1248>"
  Bus Selector23/7 -> fcn Asi Storage/7(u7)  "<Value_1258>"
  Bus Selector23/8 -> fcn Asi Storage/8(u8)  "<Value_1268>"
  Bus Selector23/9 -> fcn Asi Storage/9(u9)  "<Value_1278>"
  Bus Selector23/10 -> fcn Asi Storage/10(u10)  "<Value_1288>"
  Bus Selector23/11 -> fcn Asi Storage/11(u11)  "<Value_1298>"
  Bus Selector23/12 -> fcn Asi Storage/12(u12)  "<Value_1308>"
  Bus Selector24/1 -> MATLAB Function1/1(u1)  "<Value_1324>"
  Bus Selector24/2 -> MATLAB Function1/2(u2)  "<Value_1334>"
  Bus Selector24/3 -> MATLAB Function1/3(u3)  "<Value_1344>"
  Bus Selector24/4 -> MATLAB Function1/4(u4)  "<Value_1354>"
  Bus Selector24/5 -> MATLAB Function1/5(u5)  "<Value_1364>"
  Bus Selector25/1 -> MATLAB Function2/1(u1)  "<Value_1380>"
  Bus Selector25/2 -> MATLAB Function2/2(u2)  "<Value_1390>"
  Bus Selector25/3 -> MATLAB Function2/3(u3)  "<Value_1400>"
  Bus Selector25/4 -> MATLAB Function2/4(u4)  "<Value_1410>"
  Bus Selector25/5 -> MATLAB Function2/5(u5)  "<Value_1420>"
  Bus Selector25/6 -> MATLAB Function2/6(u6)  "<Value_1430>"
  Bus Selector25/7 -> MATLAB Function2/7(u7)  "<Value_1440>"
  Bus Selector25/8 -> MATLAB Function2/8(u8)  "<Value_1450>"
  Bus Selector26/1 -> MATLAB Function3/1(u1)  "<Value_1469>"
  Bus Selector26/2 -> MATLAB Function3/2(u2)  "<Value_1482>"
  Bus Selector26/3 -> MATLAB Function3/3(u3)  "<Value_1495>"
  Bus Selector26/4 -> MATLAB Function3/4(u4)  "<Value_1508>"
  Bus Selector26/5 -> MATLAB Function3/5(u5)  "<Value_1521>"
  Bus Selector26/6 -> MATLAB Function3/6(u6)  "<Value_1534>"
  Bus Selector26/7 -> MATLAB Function3/7(u7)  "<Value_1547>"
  Bus Selector26/8 -> MATLAB Function3/8(u8)  "<Value_1560>"
  OPC UA Read2/1 -> Bus Selector9/1, Bus Selector8/1, Bus Selector7/1
  Bus Selector7/1 -> Control1/1(u1)  "<Value_1382>"
  Bus Selector7/2 -> Control1/2(u2)  "<Value_1392>"
  Bus Selector7/3 -> Control1/3(u3)  "<Value_1402>"
  Bus Selector7/4 -> Control1/4(u4)  "<Value_1412>"
  Bus Selector7/5 -> Control1/5(u5)  "<Value_1422>"
  Bus Selector7/6 -> Control1/6(u6)  "<Value_1432>"
  Bus Selector7/7 -> Control1/7(u7)  "<Value_1442>"
  Bus Selector7/8 -> Control1/8(u8)  "<Value_1452>"
  Bus Selector7/9 -> Control1/9(u9)  "<Value_1462>"
  Bus Selector7/10 -> Control1/10(u10)  "<Value_1472>"
  Bus Selector7/11 -> Control1/11(u11)  "<Value_1482>"
  Bus Selector7/12 -> Control1/12(u12)  "<Value_1492>"
  Bus Selector7/13 -> Control1/13(u13)  "<Value_1502>"
  Bus Selector7/14 -> Control1/14(u14)  "<Value_1512>"
  Bus Selector7/15 -> Control1/15(u15)  "<Value_1522>"
  Bus Selector7/16 -> Control1/16(u16)  "<Value_1532>"
  Bus Selector7/17 -> Control1/17(u17)  "<Value_1542>"
  Bus Selector7/18 -> Control1/18(u18)  "<Value_1552>"
  Bus Selector7/19 -> Control1/19(u19)  "<Value_1562>"
  Bus Selector7/20 -> Control1/20(u20)  "<Value_1572>"
  Bus Selector7/21 -> Control1/21(u21)  "<Value_1582>"
  Bus Selector7/22 -> Control1/22(u22)  "<Value_1592>"
  Bus Selector7/23 -> Control1/23(u23)  "<Value_1602>"
  Bus Selector7/24 -> Control1/24(u24)  "<Value_1612>"
  Bus Selector8/1 -> Feedback1/1(u1)  "<Value_1628>"
  Bus Selector8/2 -> Feedback1/2(u2)  "<Value_1638>"
  Bus Selector8/3 -> Feedback1/3(u3)  "<Value_1648>"
  Bus Selector8/4 -> Feedback1/4(u4)  "<Value_1658>"
  Bus Selector8/5 -> Feedback1/5(u5)  "<Value_1668>"
  Bus Selector8/6 -> Feedback1/6(u6)  "<Value_1678>"
  Bus Selector8/7 -> Feedback1/7(u7)  "<Value_1688>"
  Bus Selector8/8 -> Feedback1/8(u8)  "<Value_1698>"
  Bus Selector8/9 -> Feedback1/9(u9)  "<Value_1708>"
  Bus Selector9/1 -> Sensors1/1(u1)  "<Value_1727>"
  Bus Selector9/2 -> Sensors1/2(u2)  "<Value_1740>"
  Bus Selector9/3 -> Sensors1/3(u3)  "<Value_1755>"
  Bus Selector9/4 -> Sensors1/4(u4)  "<Value_1768>"
  Bus Selector9/5 -> Sensors1/5(u5)  "<Value_1781>"
  Bus Selector9/6 -> Sensors1/6(u6)  "<Value_1794>"
  Bus Selector9/7 -> Sensors1/7(u7)  "<Value_1807>"
  Bus Selector9/8 -> Sensors1/8(u8)  "<Value_1820>"
  Bus Selector9/9 -> Sensors1/9(u9)  "<Value_1833>"
  Bus Selector9/10 -> Sensors1/10(u10)  "<Value_1846>"
  Bus Selector9/11 -> Sensors1/11(u11)  "<Value_1859>"
  Bus Selector9/12 -> Sensors1/12(u12)  "<Value_1872>"
  Bus Selector9/13 -> Sensors1/13(u13)  "<Value_1885>"
  Bus Selector9/14 -> Sensors1/14(u14)  "<Value_1898>"
  Bus Selector9/15 -> Sensors1/15(u15)  "<Value_1911>"
  Bus Selector9/16 -> Sensors1/16(u16)  "<Value_1924>"
  Bus Selector9/17 -> Sensors1/17(u17)  "<Value_1937>"
  Bus Selector9/18 -> Sensors1/18(u18)  "<Value_1950>"
  Bus Selector9/19 -> Sensors1/19(u19)  "<Value_1963>"
  Bus Selector9/20 -> Sensors1/20(u20)  "<Value_1976>"
  Bus Selector9/21 -> Sensors1/21(u21)  "<Value_1989>"
  Bus Selector9/22 -> Sensors1/22(u22)  "<Value_2002>"
  Bus Selector9/23 -> Sensors1/23(u23)  "<Value_2015>"
  Bus Selector9/24 -> Sensors1/24(u24)  "<Value_2028>"
  Bus Selector9/25 -> Sensors1/25(u25)  "<Value_2041>"
  Bus Selector9/26 -> Sensors1/26(u26)  "<Value_2054>"
  Bus Selector9/27 -> Sensors1/27(u27)  "<Value_2067>"
  Bus Selector9/28 -> Sensors1/28(u28)  "<Value_2080>"
  Bus Selector9/29 -> Sensors1/29(u29)  "<Value_2093>"
  Bus Selector9/30 -> Sensors1/30(u30)  "<Value_2106>"
  Bus Selector9/31 -> Sensors1/31(u31)  "<Value_2119>"
  Bus Selector9/32 -> Sensors1/32(u32)  "<Value_2132>"
  Bus Selector9/33 -> Sensors1/33(u33)  "<Value_2145>"
  OPC UA Read/1 -> Bus Selector2/1, Bus Selector1/1, Bus Selector/1
  OPC UA Read1/1 -> Bus Selector6/1, Bus Selector5/1, Bus Selector3/1, Bus Selector4/1
  OPC UA Read5/1 -> Bus Selector27/1, Bus Selector29/1, Bus Selector28/1
  OPC UA Read7/1 -> Bus Selector20/1, Bus Selector21/1, Bus Selector22/1
  OPC UA Read3/1 -> Bus Selector10/1
  Bus Selector3/1 -> ASI/1(u1)  "<Value_1455>"
  Bus Selector3/2 -> ASI/2(u2)  "<Value_1465>"
  Bus Selector3/3 -> ASI/3(u3)  "<Value_1475>"
  Bus Selector3/4 -> ASI/4(u4)  "<Value_1485>"
  Bus Selector3/5 -> ASI/5(u5)  "<Value_1495>"
  Bus Selector3/6 -> ASI/6(u6)  "<Value_1505>"
  Bus Selector3/7 -> ASI/7(u7)  "<Value_1515>"
  Bus Selector3/8 -> ASI/8(u8)  "<Value_1525>"
  Bus Selector3/9 -> ASI/9(u9)  "<Value_1535>"
  Bus Selector3/10 -> ASI/10(u10)  "<Value_1545>"
  Bus Selector3/11 -> ASI/11(u11)  "<Value_1555>"
  Bus Selector3/12 -> ASI/12(u12)  "<Value_1565>"
  Bus Selector3/13 -> ASI/13(u13)  "<Value_1575>"
  Bus Selector4/1 -> Control/1(u1)  "<Value_1591>"
  Bus Selector4/2 -> Control/2(u2)  "<Value_1601>"
  Bus Selector4/3 -> Control/3(u3)  "<Value_1611>"
  Bus Selector4/4 -> Control/4(u4)  "<Value_1621>"
  Bus Selector4/5 -> Control/5(u5)  "<Value_1631>"
  Bus Selector4/6 -> Control/6(u6)  "<Value_1641>"
  Bus Selector4/7 -> Control/7(u7)  "<Value_1651>"
  Bus Selector4/8 -> Control/8(u8)  "<Value_1661>"
  Bus Selector4/9 -> Control/9(u9)  "<Value_1671>"
  Bus Selector4/10 -> Control/10(u10)  "<Value_1681>"
  Bus Selector4/11 -> Control/11(u11)  "<Value_1691>"
  Bus Selector4/12 -> Control/12(u12)  "<Value_1701>"
  Bus Selector4/13 -> Control/13(u13)  "<Value_1711>"
  controls/1(C_85_Initialization) -> Bus Creator/1
  controls/2(C_85_Part_Del) -> Bus Creator/2
  controls/3(C_85_Part_Mag) -> Bus Creator/3
  controls/4(C_86_Mag_Parts) -> Bus Creator/4
  controls/5(C_87_RQ_MParts) -> Bus Creator/5
  controls/6(C_82_Profibus) -> Bus Creator/6
  controls/7(C_83_RQ_Parts) -> Bus Creator/7
  controls/8(C_85_Start) -> Bus Creator/8
  controls/9(C_85_Single) -> Bus Creator/9
  controls/10(C_85_Continuous) -> Bus Creator/10
  controls/11(C_85_Counted) -> Bus Creator/11
  Bus Selector1/1 -> feedback/1(u1)  "<Value_1317>"
  Bus Selector1/2 -> feedback/2(u2)  "<Value_1327>"
  Bus Selector1/3 -> feedback/3(u3)  "<Value_1337>"
  Bus Selector1/4 -> feedback/4(u4)  "<Value_1347>"
  Bus Selector1/5 -> feedback/5(u5)  "<Value_1357>"
  Bus Selector1/6 -> feedback/6(u6)  "<Value_1367>"
  Bus Selector1/7 -> feedback/7(u7)  "<Value_1377>"
  Bus Selector1/8 -> feedback/8(u8)  "<Value_1387>"
  Bus Selector1/9 -> feedback/9(u9)  "<Value_1397>"
  Bus Selector1/10 -> feedback/10(u10)  "<Value_1407>"
  Bus Selector1/11 -> feedback/11(u11)  "<Value_1417>"
  Bus Selector1/12 -> feedback/12(u12)  "<Value_1427>"
  Bus Selector1/13 -> feedback/13(u13)  "<Value_1437>"
  Bus Selector/1 -> controls/1(u1)  "<Value_1195>"
  Bus Selector/2 -> controls/2(u2)  "<Value_1205>"
  Bus Selector/3 -> controls/3(u3)  "<Value_1215>"
  Bus Selector/4 -> controls/4(u4)  "<Value_1227>"
  Bus Selector/5 -> controls/5(u5)  "<Value_1239>"
  Bus Selector/6 -> controls/6(u6)  "<Value_1249>"
  Bus Selector/7 -> controls/7(u7)  "<Value_1261>"
  Bus Selector/8 -> controls/8(u8)  "<Value_1271>"
  Bus Selector/9 -> controls/9(u9)  "<Value_1281>"
  Bus Selector/10 -> controls/10(u10)  "<Value_1291>"
  Bus Selector/11 -> controls/11(u11)  "<Value_1301>"
  Bus Selector2/1 -> sensors/1(u1)  "<Value_1458>"
  Bus Selector2/2 -> sensors/2(u2)  "<Value_1471>"
  Bus Selector2/3 -> sensors/3(u3)  "<Value_1486>"
  Bus Selector2/4 -> sensors/4(u4)  "<Value_1499>"
  Bus Selector2/5 -> sensors/5(u5)  "<Value_1512>"
  Bus Selector2/6 -> sensors/6(u6)  "<Value_1525>"
  Bus Selector2/7 -> sensors/7(u7)  "<Value_1538>"
  Bus Selector2/8 -> sensors/8(u8)  "<Value_1551>"
  Bus Selector2/9 -> sensors/9(u9)  "<Value_1564>"
  Bus Selector2/10 -> sensors/10(u10)  "<Value_1577>"
  Bus Selector2/11 -> sensors/11(u11)  "<Value_1590>"
  Bus Selector2/12 -> sensors/12(u12)  "<Value_1603>"
  Bus Selector2/13 -> sensors/13(u13)  "<Value_1616>"
  Bus Selector2/14 -> sensors/14(u14)  "<Value_1629>"
  Bus Selector2/15 -> sensors/15(u15)  "<Value_1642>"
  Bus Selector6/1 -> Sensors/1(u1)  "<Value_1858>"
  Bus Selector6/2 -> Sensors/2(u2)  "<Value_1871>"
  Bus Selector6/3 -> Sensors/3(u3)  "<Value_1886>"
  Bus Selector6/4 -> Sensors/4(u4)  "<Value_1899>"
  Bus Selector6/5 -> Sensors/5(u5)  "<Value_1912>"
  Bus Selector6/6 -> Sensors/6(u6)  "<Value_1925>"
  Bus Selector6/7 -> Sensors/7(u7)  "<Value_1938>"
  Bus Selector6/8 -> Sensors/8(u8)  "<Value_1951>"
  Bus Selector6/9 -> Sensors/9(u9)  "<Value_1964>"
  Bus Selector6/10 -> Sensors/10(u10)  "<Value_1977>"
  Bus Selector6/11 -> Sensors/11(u11)  "<Value_1990>"
  Bus Selector6/12 -> Sensors/12(u12)  "<Value_2003>"
  Bus Selector6/13 -> Sensors/13(u13)  "<Value_2016>"
  Bus Selector6/14 -> Sensors/14(u14)  "<Value_2029>"
  Bus Selector6/15 -> Sensors/15(u15)  "<Value_2042>"
  Bus Selector5/1 -> Feedback/1(u1)  "<Value_1727>"
  Bus Selector5/2 -> Feedback/2(u2)  "<Value_1737>"
  Bus Selector5/3 -> Feedback/3(u3)  "<Value_1747>"
  Bus Selector5/4 -> Feedback/4(u4)  "<Value_1757>"
  Bus Selector5/5 -> Feedback/5(u5)  "<Value_1767>"
  Bus Selector5/6 -> Feedback/6(u6)  "<Value_1777>"
  Bus Selector5/7 -> Feedback/7(u7)  "<Value_1787>"
  Bus Selector5/8 -> Feedback/8(u8)  "<Value_1797>"
  Bus Selector5/9 -> Feedback/9(u9)  "<Value_1807>"
  Bus Selector5/10 -> Feedback/10(u10)  "<Value_1817>"
  Bus Selector5/11 -> Feedback/11(u11)  "<Value_1827>"
  Bus Selector5/12 -> Feedback/12(u12)  "<Value_1837>"
  Bus Selector27/1 -> Control4/1(u1)  "<Value_1204>"
  Bus Selector27/2 -> Control4/2(u2)  "<Value_1214>"
  Bus Selector27/3 -> Control4/3(u3)  "<Value_1224>"
  Bus Selector27/4 -> Control4/4(u4)  "<Value_1234>"
  Bus Selector27/5 -> Control4/5(u5)  "<Value_1244>"
  Bus Selector27/6 -> Control4/6(u6)  "<Value_1254>"
  Bus Selector27/7 -> Control4/7(u7)  "<Value_1264>"
  Bus Selector27/8 -> Control4/8(u8)  "<Value_1274>"
  Bus Selector27/9 -> Control4/9(u9)  "<Value_1284>"
  Bus Selector27/10 -> Control4/10(u10)  "<Value_1294>"
  Bus Selector28/1 -> Feedback4/1(u1)  "<Value_1310>"
  Bus Selector28/2 -> Feedback4/2(u2)  "<Value_1320>"
  Bus Selector28/3 -> Feedback4/3(u3)  "<Value_1330>"
  Bus Selector28/4 -> Feedback4/4(u4)  "<Value_1340>"
  Bus Selector28/5 -> Feedback4/5(u5)  "<Value_1350>"
  Bus Selector28/6 -> Feedback4/6(u6)  "<Value_1360>"
  Bus Selector28/7 -> Feedback4/7(u7)  "<Value_1370>"
  Bus Selector28/8 -> Feedback4/8(u8)  "<Value_1380>"
  Bus Selector28/9 -> Feedback4/9(u9)  "<Value_1390>"
  Bus Selector28/10 -> Feedback4/10(u10)  "<Value_1400>"
  Bus Selector28/11 -> Feedback4/11(u11)  "<Value_1410>"
  Bus Selector28/12 -> Feedback4/12(u12)  "<Value_1420>"
  Bus Selector28/13 -> Feedback4/13(u13)  "<Value_1430>"
  Bus Selector28/14 -> Feedback4/14(u14)  "<Value_1440>"
  Bus Selector29/1 -> Sensors4/1(u1)  "<Value_1461>"
  Bus Selector29/2 -> Sensors4/2(u2)  "<Value_1474>"
  Bus Selector29/3 -> Sensors4/3(u3)  "<Value_1489>"
  Bus Selector29/4 -> Sensors4/4(u4)  "<Value_1502>"
  Bus Selector29/5 -> Sensors4/5(u5)  "<Value_1515>"
  Bus Selector29/6 -> Sensors4/6(u6)  "<Value_1528>"
  Bus Selector29/7 -> Sensors4/7(u7)  "<Value_1541>"
  Bus Selector29/8 -> Sensors4/8(u8)  "<Value_1554>"
  Bus Selector29/9 -> Sensors4/9(u9)  "<Value_1567>"
  Bus Selector29/10 -> Sensors4/10(u10)  "<Value_1580>"
  Bus Selector29/11 -> Sensors4/11(u11)  "<Value_1593>"
  Bus Selector29/12 -> Sensors4/12(u12)  "<Value_1606>"
  Bus Selector29/13 -> Sensors4/13(u13)  "<Value_1619>"
  Bus Selector29/14 -> Sensors4/14(u14)  "<Value_1632>"
  Bus Selector29/15 -> Sensors4/15(u15)  "<Value_1645>"
  Bus Selector20/1 -> Control5/1(u1)  "<Value_1178>"
  Bus Selector20/2 -> Control5/2(u2)  "<Value_1188>"
  Bus Selector20/3 -> Control5/3(u3)  "<Value_1198>"
  Bus Selector20/4 -> Control5/4(u4)  "<Value_1208>"
  Bus Selector20/5 -> Control5/5(u5)  "<Value_1218>"
  Bus Selector20/6 -> Control5/6(u6)  "<Value_1228>"
  Bus Selector20/7 -> Control5/7(u7)  "<Value_1238>"
  Bus Selector20/8 -> Control5/8(u8)  "<Value_1248>"
  Bus Selector20/9 -> Control5/9(u9)  "<Value_1258>"
  Bus Selector20/10 -> Control5/10(u10)  "<Value_1268>"
  Bus Selector20/11 -> Control5/11(u11)  "<Value_1278>"
  Bus Selector21/1 -> Feedback5/1(u1)  "<Value_1294>"
  Bus Selector21/2 -> Feedback5/2(u2)  "<Value_1304>"
  Bus Selector21/3 -> Feedback5/3(u3)  "<Value_1314>"
  Bus Selector21/4 -> Feedback5/4(u4)  "<Value_1324>"
  Bus Selector21/5 -> Feedback5/5(u5)  "<Value_1334>"
  Bus Selector21/6 -> Feedback5/6(u6)  "<Value_1344>"
  Bus Selector21/7 -> Feedback5/7(u7)  "<Value_1354>"
  Bus Selector21/8 -> Feedback5/8(u8)  "<Value_1364>"
  Bus Selector21/9 -> Feedback5/9(u9)  "<Value_1374>"
  Bus Selector21/10 -> Feedback5/10(u10)  "<Value_1384>"
  Bus Selector21/11 -> Feedback5/11(u11)  "<Value_1394>"
  Bus Selector21/12 -> Feedback5/12(u12)  "<Value_1404>"
  Bus Selector22/1 -> Sensors5/1(u1)  "<Value_1423>"
  Bus Selector22/2 -> Sensors5/2(u2)  "<Value_1436>"
  Bus Selector22/3 -> Sensors5/3(u3)  "<Value_1451>"
  Bus Selector22/4 -> Sensors5/4(u4)  "<Value_1464>"
  Bus Selector22/5 -> Sensors5/5(u5)  "<Value_1477>"
  Bus Selector22/6 -> Sensors5/6(u6)  "<Value_1490>"
  Bus Selector22/7 -> Sensors5/7(u7)  "<Value_1503>"
  Bus Selector22/8 -> Sensors5/8(u8)  "<Value_1516>"
  Bus Selector22/9 -> Sensors5/9(u9)  "<Value_1529>"
  Bus Selector22/10 -> Sensors5/10(u10)  "<Value_1542>"
  Bus Selector22/11 -> Sensors5/11(u11)  "<Value_1555>"
  Bus Selector22/12 -> Sensors5/12(u12)  "<Value_1568>"
  Bus Selector22/13 -> Sensors5/13(u13)  "<Value_1581>"
  Bus Selector22/14 -> Sensors5/14(u14)  "<Value_1594>"
  Bus Selector22/15 -> Sensors5/15(u15)  "<Value_1607>"
  Bus Selector22/16 -> Sensors5/16(u16)  "<Value_1620>"
  Bus Selector10/1 -> Asi/1(u1)  "<Value_1457>"
  Bus Selector10/2 -> Asi/2(u2)  "<Value_1467>"
  Bus Selector10/3 -> Asi/3(u3)  "<Value_1477>"
  Bus Selector10/4 -> Asi/4(u4)  "<Value_1487>"
  Bus Selector10/5 -> Asi/5(u5)  "<Value_1497>"
  Bus Selector10/6 -> Asi/6(u6)  "<Value_1507>"
  Bus Selector10/7 -> Asi/7(u7)  "<Value_1517>"
  Bus Selector10/8 -> Asi/8(u8)  "<Value_1527>"
  Bus Selector10/9 -> Asi/9(u9)  "<Value_1537>"
  Bus Selector10/10 -> Asi/10(u10)  "<Value_1547>"
  Bus Selector10/11 -> Asi/11(u11)  "<Value_1557>"
  Bus Selector10/12 -> Asi/12(u12)  "<Value_1567>"
  Asi/1(A_54_Request) -> Bus Creator10/1
  Asi/2(A_54_No_Cart) -> Bus Creator10/2
  Asi/3(A_54_Cart_Full) -> Bus Creator10/3
  Asi/4(A_54_CRoute_Out) -> Bus Creator10/4
  Asi/5(A_53_SortCartID) -> Bus Creator10/5
  Asi/6(A_54_Cart_Stat) -> Bus Creator10/6
  Asi/7(A_54_Cart_Next) -> Bus Creator10/7
  Asi/8(A_54_Optic) -> Bus Creator10/8
  Asi/9(A_54_Count) -> Bus Creator10/9
  Asi/10(A_54_Pist_Bck) -> Bus Creator10/10
  Asi/11(A_54_Release_FB) -> Bus Creator10/11
  Asi/12(A_54_CRoute_In) -> Bus Creator10/12
